simulink subsystem "Lazo_Torque"  (R2026a)
settings: Solver=VariableStepAuto
values from neighbouring files (symbols this model uses):
  k_l = 0.1    [coeficientes.m]
  L_d = 6.6e-3    (= 0.0066)    [coeficientes.m]
  L_q = 5.8e-3    (= 0.0058)    [coeficientes.m]
  lambda = 0.016    [coeficientes.m]
  Pp = 3    [coeficientes.m]
  r_m2l = 120.0    (= 120)    [coeficientes.m]
libraries: eeTransforms x1
settings Model: Creator=admin  LastModifiedBy=admin

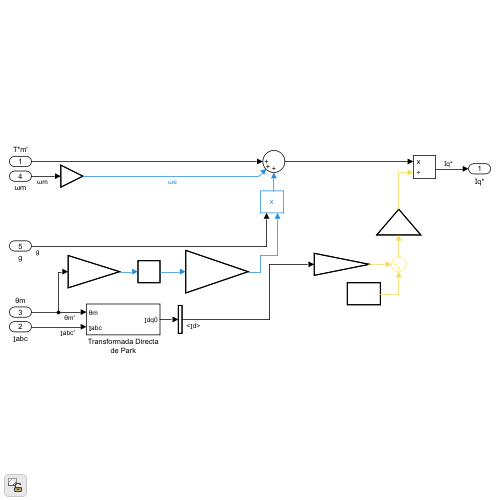
[thumbnail: Simulink's stored preview of the top-level diagram]
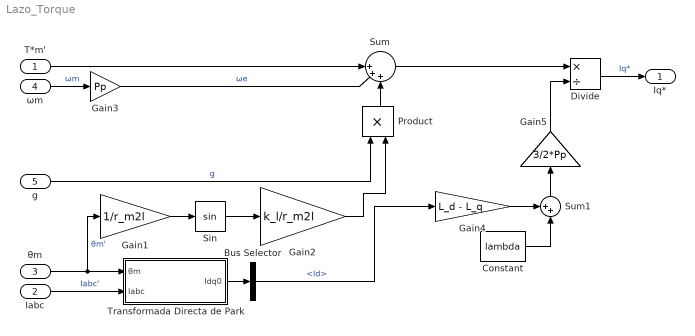
== system Lazo_Torque ==
  T*m' : Inport
  Ⅰabc : Inport  Port=2
  θm : Inport  Port=3
  ωm : Inport  Port=4
  g : Inport  Port=5
  Bus Selector : BusSelector  OutputSignals=Ⅰd
  Constant : Constant  Value=lambda
  Divide : Product  Inputs=*/
  Gain1 : Gain  Gain=1/r_m2l
  Gain2 : Gain  Gain=k_l/r_m2l
  Gain3 : Gain  Gain=Pp
  Gain4 : Gain  Gain=L_d - L_q
  Gain5 : Gain  Gain=3/2*Pp
  Product : Product
  Sin : Trigonometry
  Sum : Sum  Inputs=||+++
  Sum1 : Sum  Inputs=++|
  Transformada Directa de Park : Subsystem
  Ⅰq* : Outport
  wires:
  Divide/1 -> Ⅰq*/1  "Ⅰq*"
  T*m'/1 -> Sum/1
  Ⅰabc/1 -> Transformada Directa de Park/2(Ⅰabc)  "Ⅰabc'"
  θm/1 -> Transformada Directa de Park/1(θm), Gain1/1  "θm'"
  Transformada Directa de Park/1(Ⅰdq0) -> Bus Selector/1
  Gain4/1 -> Sum1/1
  Constant/1 -> Sum1/2
  Sum1/1 -> Gain5/1
  Sum/1 -> Divide/1
  Gain5/1 -> Divide/2
  Bus Selector/1 -> Gain4/1  "<Ⅰd>"
  Gain1/1 -> Sin/1
  Sin/1 -> Gain2/1
  Product/1 -> Sum/3
  Gain2/1 -> Product/2
  g/1 -> Product/1  "g"
  ωm/1 -> Gain3/1  "ωm"
  Gain3/1 -> Sum/2  "ωe"

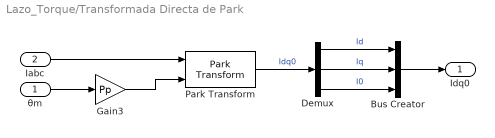
== system Lazo_Torque/Transformada Directa de Park ==
  θm : Inport
  Ⅰabc : Inport  Port=2
  Bus Creator : BusCreator  Inputs=3
  Demux : Demux  Outputs=3
  Gain3 : Gain  Gain=Pp
  Park Transform : eeTransforms/Park Transform  AxisAlignment=Q-axis  PowerInvariant=off
      settings: LibrarySourceBlock=|
      | ee_sl_lib/Mathematical
      | Transforms/Park Transform
  Ⅰdq0 : Outport
  wires:
  Gain3/1 -> Park Transform/2
  Park Transform/1 -> Demux/1  "Ⅰdq0"
  Demux/1 -> Bus Creator/1  "Ⅰd"
  Demux/3 -> Bus Creator/3  "Ⅰ0"
  Demux/2 -> Bus Creator/2  "Ⅰq"
  Bus Creator/1 -> Ⅰdq0/1
  Ⅰabc/1 -> Park Transform/1
  θm/1 -> Gain3/1
